simulink model "SlottingModel"  (Simulink 7.9)
settings: Solver=VariableStepDiscrete  StartTime=0.0  StopTime=100.0  RelTol=1e-3
settings Model: Creator=tsprock3  LastModifiedBy=tsprock3
settings DebuggingCC: SimStateOlderReleaseMsg=warning

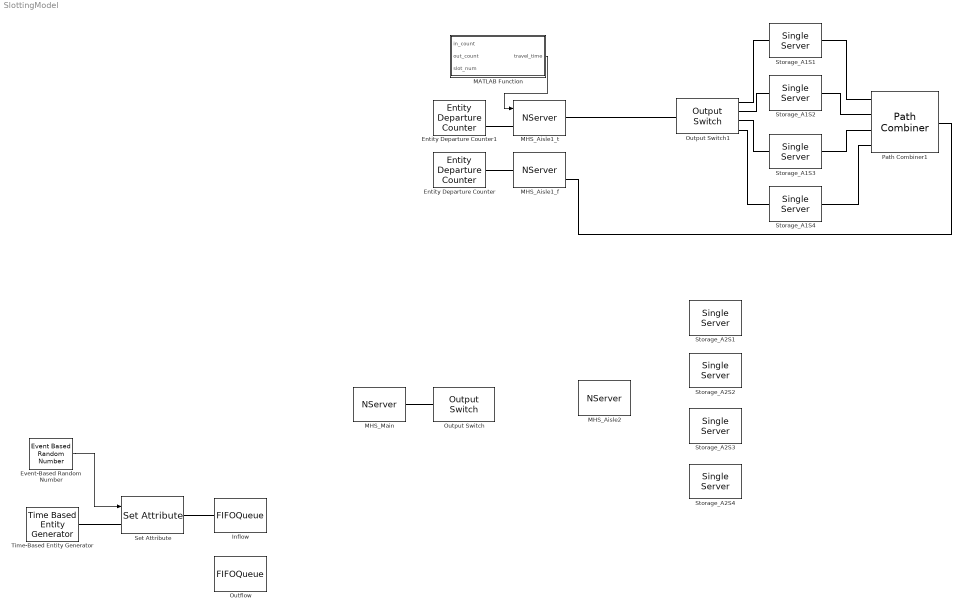
== system SlottingModel ==
  Entity Departure Counter : EntityDepartureCounter  NumberDepartedToSignal=on  NumberDepartedToAttribute=off
  Entity Departure Counter1 : EntityDepartureCounter  NumberDepartedToSignal=on  NumberDepartedToAttribute=off
  Event-Based Random Number : EventBasedRandomNumber  Distribution=Arbitrary discrete  valueVecDisc=[1 2]
  Inflow : FIFOQueue
  MATLAB Function : MATLAB Function  TreatAsAtomicUnit=on
  MHS_Aisle1_f : NServer  NumberOfServers=inf  ServiceTimeFrom=Signal port t
  MHS_Aisle1_t : NServer  NumberOfServers=inf  ServiceTimeFrom=Signal port t
  MHS_Aisle2 : NServer
  MHS_Main : NServer
  Outflow : FIFOQueue
  Output Switch : OutputSwitch
  Output Switch1 : OutputSwitch  NumberOutputPorts=4  SwitchingCriterion=From attribute  AttributeName=Slot
  Path Combiner1 : PathCombiner  NumberInputPorts=4
  Set Attribute : SetAttribute  AttributeName=Product|Creation_Time|Putaway_Start|Putaway_End|Aisle|Slot  AttributeFrom=Signal port|Dialog|Dialog|Dialog|Dialog|Dialog  AttributeValue=1|1|1|1|1|1  AttributeTreatAsVector=1|1|1|1|1|1  EvaluatedAttributeValue={[];1;1;1;1;1}
  Storage_A1S{1..4} (4 alike) : SingleServer
  Storage_A2S{1..4} (4 alike) : SingleServer
  Time-Based Entity Generator : TimeBasedEntityGenerator
  wires:
  Event-Based Random Number/1 -> Set Attribute/1
  MATLAB Function/1(travel_time) -> MHS_Aisle1_t/1
  connections:
  Time-Based Entity Generator/RConn1 -- Set Attribute/LConn1
  Set Attribute/RConn1 -- Inflow/LConn1
  MHS_Main/RConn1 -- Output Switch/LConn1
  Output Switch1/RConn1 -- Storage_A1S1/LConn1
  Output Switch1/RConn2 -- Storage_A1S2/LConn1
  Output Switch1/RConn3 -- Storage_A1S3/LConn1
  Output Switch1/RConn4 -- Storage_A1S4/LConn1
  Storage_A1S1/RConn1 -- Path Combiner1/LConn1
  Storage_A1S2/RConn1 -- Path Combiner1/LConn2
  Storage_A1S3/RConn1 -- Path Combiner1/LConn3
  Storage_A1S4/RConn1 -- Path Combiner1/LConn4
  Path Combiner1/RConn1 -- MHS_Aisle1_f/LConn1
  MHS_Aisle1_t/RConn1 -- Output Switch1/LConn1
  Entity Departure Counter/LConn1 -- MHS_Aisle1_f/RConn1
  Entity Departure Counter1/RConn1 -- MHS_Aisle1_t/LConn1

== matlab function MATLAB Function ==
  data: in_count input double; travel_time output double; out_count input double; slot_num input double
function travel_time = fcn(in_count, out_count, slot_num)
%#codegen

travel_time = 0.25*slot_num;
